simulink model "Quadcopter_State_model_Arduino"  (R2023b)
settings: Solver=VariableStepAuto  StartTime=0.0  StopTime=inf  FixedStep=0.00001  MinStep=0.001  RelTol=1e-3
model workspace (MAT data in the model file):
  DesiredPitchRoll : sugfis (value not decoded)
  DesiredThrust : sugfis (value not decoded)
  DesiredYaw : sugfis (value not decoded)
  Desired_Pitch = 0
  Desired_Roll = 0
  Desired_Yaw = 0
  Desired_Z_Velocity = -3
  FuzzyMotorspeed : sugfis (value not decoded)
values from neighbouring files (symbols this model uses):
  g = 9.81    [Quadcopter_Constants.m]
  Ixx = 0.0294838    [Quadcopter_Constants.m]
  Iyy = 0.0294838    [Quadcopter_Constants.m]
  Izz = 0.058967624    [Quadcopter_Constants.m]
  Jr = (6e-5)*1.358    (= 8.148e-05)    [Quadcopter_Constants.m]
  kd = 1    [Quadcopter_Constants.m]
  kd_phi = 1    [Quadcopter_Constants.m]
  kd_theta = 1    [Quadcopter_Constants.m]
  kf = 1    [Quadcopter_Constants.m]
  ki = 1    [Quadcopter_Constants.m]
  ki_phi = 1    [Quadcopter_Constants.m]
  ki_theta = 1    [Quadcopter_Constants.m]
  km = 4.74157e-9    (= 4.74157e-09)    [Quadcopter_Constants.m]
  kp = 1    [Quadcopter_Constants.m]
  kp_phi = 1    [Quadcopter_Constants.m]
  kp_theta = 1    [Quadcopter_Constants.m]
  kr = (0.1)*1.358    (= 0.1358)    [Quadcopter_Constants.m]
  kt = (0.1)*1.358    (= 0.1358)    [Quadcopter_Constants.m]
  l = 0.254    [Quadcopter_Constants.m]
  m = 0.914    [Quadcopter_Constants.m]
  sample_freq = 1000    [Quadcopter_Constants.m]
undefined symbols (not defined in the file or in its folder): LF
libraries: fuzblock x18, instrumentseriallib x12, simulink_extras x6, vrlib x4, instrumentlib x3, etargetslib x1, slpidlib x1, simulink x1
(part 3 of 5)

== system Quadcopter_State_model_Arduino/Arduino Sim/Control Vector ==
  Omega_1 : Inport
  Omega_2 : Inport  Port=2
  Omega_3 : Inport  Port=3
  Omega_4 : Inport  Port=4
  Constant : Constant  Value=kf
  Constant1 : Constant  Value=km
  Product{,1..3} (4 alike) : Product
  Square{,1..3} (4 alike) : Math  Operator=square
  Sum : Sum  Inputs=++++
  Sum1 : Sum  Inputs=-+
  Sum2 : Sum  Inputs=+-
  Sum3 : Sum  Inputs=+-+-
  U1 : Outport
  U2 : Outport  Port=2
  U3 : Outport  Port=3
  U4 : Outport  Port=4
  wires:
  Omega_1/1 -> Square/1
  Omega_2/1 -> Square1/1
  Omega_3/1 -> Square2/1
  Omega_4/1 -> Square3/1
  Constant/1 -> Product2/2, Product1/2, Product/2
  Sum/1 -> Product/1
  Product/1 -> U1/1
  Square/1 -> Sum3/1, Sum2/1, Sum/1
  Square1/1 -> Sum3/2, Sum1/1, Sum/2
  Square2/1 -> Sum3/3, Sum2/2, Sum/3
  Square3/1 -> Sum1/2, Sum/4, Sum3/4
  Sum1/1 -> Product1/1
  Product1/1 -> U2/1
  Sum2/1 -> Product2/1
  Product2/1 -> U3/1
  Constant1/1 -> Product3/2
  Sum3/1 -> Product3/1
  Product3/1 -> U4/1

== system Quadcopter_State_model_Arduino/Arduino Sim/Quadcopter Dynamics1 ==
  U1 : Inport
  U2 : Inport  Port=2
  U3 : Inport  Port=3
  U4 : Inport  Port=4
  Omega_R : Inport  Port=5
  Bus Creator : BusCreator  Inputs=12
  Rotational Subsystem : Subsystem
  Translational Subsystem 2.0 : Subsystem
  Translational Wind Engine : Subsystem
  X_State : Outport
  wires:
  Rotational Subsystem/5(psi) -> Translational Subsystem 2.0/4(psi), Translational Wind Engine/3(psi), Bus Creator/5  "psi"
  Rotational Subsystem/2(phi_dot) -> Bus Creator/2  "phi_dot"
  Rotational Subsystem/3(theta) -> Translational Subsystem 2.0/3(theta), Translational Wind Engine/2(theta), Bus Creator/3  "theta"
  Rotational Subsystem/1(phi) -> Translational Subsystem 2.0/2(phi), Translational Wind Engine/1(phi), Bus Creator/1  "phi"
  Rotational Subsystem/4(theta_dot) -> Bus Creator/4  "theta_dot"
  Bus Creator/1 -> X_State/1  "X_State"
  Rotational Subsystem/6(psi_dot) -> Bus Creator/6  "psi_dot"
  U4/1 -> Rotational Subsystem/3(U4)
  U3/1 -> Rotational Subsystem/2(U3)
  U2/1 -> Rotational Subsystem/1(U2)
  Omega_R/1 -> Rotational Subsystem/4(Omega_R)
  Translational Wind Engine/1(FWx) -> Translational Subsystem 2.0/5(FWx)
  Translational Wind Engine/2(FWy) -> Translational Subsystem 2.0/6(FWy)
  Translational Wind Engine/3(FWz) -> Translational Subsystem 2.0/7(FWz)
  U1/1 -> Translational Subsystem 2.0/1(U1)
  Translational Subsystem 2.0/1(x) -> Bus Creator/7  "x"
  Translational Subsystem 2.0/2(x_dot) -> Bus Creator/8  "x_dot"
  Translational Subsystem 2.0/3(y) -> Bus Creator/9  "y"
  Translational Subsystem 2.0/4(y_dot) -> Bus Creator/10  "y_dot"
  Translational Subsystem 2.0/5(z) -> Bus Creator/11  "z"
  Translational Subsystem 2.0/6(z_dot) -> Bus Creator/12  "z_dot"

== system Quadcopter_State_model_Arduino/Arduino Sim/Relative Speed ==
  Omega_1 : Inport
  Omega_2 : Inport  Port=2
  Omega_3 : Inport  Port=3
  Omega_4 : Inport  Port=4
  Add4 : Sum  Inputs=-+-+
  Omega_R : Outport
  wires:
  Omega_1/1 -> Add4/1
  Add4/1 -> Omega_R/1  "Omega_R"
  Omega_2/1 -> Add4/2
  Omega_3/1 -> Add4/3
  Omega_4/1 -> Add4/4

== system Quadcopter_State_model_Arduino/Arduino Sim/Visualization ==
  X_State : Inport
  Bus Creator1 : BusCreator  Inputs=3
  Bus Selector1 : BusSelector  OutputSignals=phi,phi_dot,theta,theta_dot,psi,psi_dot,x,x_dot,y,y_dot,z,z_dot
  Gain : Gain
  Gain1 : Gain  Gain=-1
  Gain2 : Gain
  Gain3 : Gain  Gain=-1
  Gain4 : Gain  Gain=-1
  Inertal to body frame : MATLAB Function  TreatAsAtomicUnit=on
  Rotation Matrix to VRML Rotation1 : vrlib/Utilities/Rotation Matrix to VR Rotation  maxzero=1e-12
  VR Sink : vrlib/VR Sink  InstantiateOnLoad=on  SampleTime=0.1  ViewEnable=on  RemoteChange=off  RemoteView=off  FieldsWritten=Wall_Mat.diffuseColor.3.1.1.double#Window_Mat.transparency.1.1.1.double#Landing_Mat.diffuseColor.3.1.1.double#Pole_1.Color.3.1.1.double#UAV.rotation.4.1.1.double#UAV.translation.3.1.1.double#HUDText1.string.1.-1.1.char  WorldFileName=uav_scene_drone_example.wrl  WorldDescription=UAV Competition Scene  AutoView=off  VideoDimensions=[]  AllowVariableSize=off  FigureProperties=[]
  wires:
  Bus Selector1/4 -> ?  "<theta_dot>"
  Bus Selector1/10 -> ?  "<y_dot>"
  X_State/1 -> Bus Selector1/1
  Bus Creator1/1 -> VR Sink/6  "X_State"
  Bus Selector1/2 -> ?  "<phi_dot>"
  Inertal to body frame/1(R) -> Rotation Matrix to VRML Rotation1/1
  ? -> VR Sink/7
  Rotation Matrix to VRML Rotation1/1 -> VR Sink/5
  ? -> VR Sink/4
  Bus Selector1/6 -> ?  "<psi_dot>"
  Bus Selector1/8 -> ?  "<x_dot>"
  Bus Selector1/12 -> ?  "<z_dot>"
  ? -> VR Sink/1
  ? -> VR Sink/2
  ? -> VR Sink/3
  Bus Selector1/11 -> Gain1/1  "<z>"
  Bus Selector1/9 -> Gain/1  "<y>"
  Bus Selector1/3 -> Gain3/1  "<theta>"
  Bus Selector1/5 -> Gain4/1  "<psi>"
  Bus Selector1/1 -> Inertal to body frame/3(psi)  "<phi>"
  Gain/1 -> Bus Creator1/1
  Gain1/1 -> Bus Creator1/2
  Bus Selector1/7 -> Gain2/1  "<x>"
  Gain2/1 -> Bus Creator1/3
  Gain3/1 -> Inertal to body frame/1(phi)
  Gain4/1 -> Inertal to body frame/2(theta)

== system Quadcopter_State_model_Arduino/Board Fuzzy Only/Control Vector ==
  Omega_1 : Inport
  Omega_2 : Inport  Port=2
  Omega_3 : Inport  Port=3
  Omega_4 : Inport  Port=4
  Constant : Constant  Value=kf
  Constant1 : Constant  Value=km
  Product{,1..3} (4 alike) : Product
  Square{,1..3} (4 alike) : Math  Operator=square
  Sum : Sum  Inputs=++++
  Sum1 : Sum  Inputs=-+
  Sum2 : Sum  Inputs=+-
  Sum3 : Sum  Inputs=+-+-
  U1 : Outport
  U2 : Outport  Port=2
  U3 : Outport  Port=3
  U4 : Outport  Port=4
  wires:
  Omega_1/1 -> Square/1
  Omega_2/1 -> Square1/1
  Omega_3/1 -> Square2/1
  Omega_4/1 -> Square3/1
  Constant/1 -> Product2/2, Product1/2, Product/2
  Sum/1 -> Product/1
  Product/1 -> U1/1
  Square/1 -> Sum3/1, Sum2/1, Sum/1
  Square1/1 -> Sum3/2, Sum1/1, Sum/2
  Square2/1 -> Sum3/3, Sum2/2, Sum/3
  Square3/1 -> Sum1/2, Sum/4, Sum3/4
  Sum1/1 -> Product1/1
  Product1/1 -> U2/1
  Sum2/1 -> Product2/1
  Product2/1 -> U3/1
  Constant1/1 -> Product3/2
  Sum3/1 -> Product3/1
  Product3/1 -> U4/1

== system Quadcopter_State_model_Arduino/Board Fuzzy Only/Fuzzy Control System ==
  note: Outputs are also mapped to a unsigned
      | 8-bit integer range. [0,255] This can be
      | scaled with a gain block or my changing
      | the FIS parameters.
  note: Here the inputs are mapped to an 8-bit integer currently.
      | Thrust: [0,255]
      | Roll: [-128,127]
      | Pitch: [-128,127]
      | Yaw: [-128,127]
      | While these are controlled by sliders currently they
      | could be controlled by a user using twin analog joysticks
      | or by another intelligent system directing flight.
      | To make a system that balances itself we could use
      | readings off the 9-axis gyro to inform the system to
      | lean in the opposite direction.
  x_state : Inport
  Attitude Controller : Subsystem
  Bus Creator : BusCreator  Inputs=4
  Bus Selector1 : BusSelector  OutputSignals=phi,phi_dot,theta,theta_dot,psi,psi_dot,x,x_dot,y,y_dot,z,z_dot
  Heading Controller : Subsystem
  Motorspeeds : fuzblock/Fuzzy Logic  Controller  FIS=FuzzyMotorspeed  OutputSampleNumber=101  DataType=double  FuzzifiedInputs=off  RuleFiringStrengths=off  RuleOutputs=off  AggregatedOutputs=off  SimulateUsing=Interpreted execution  OutOfRangeInputValueMessage=warning  NoRuleFiredMessage=warning  EmptyOutputFuzzySetMessage=warning
  Saturation1 : Saturate  UpperLimit=255  LowerLimit=0  OutMin=[0]  OutMax=[255]
  Scope4 : Scope  NumInputPorts=4
  Thrust Controller : Subsystem
  motorspeeds : Outport
  wires:
  Motorspeeds/1 -> motorspeeds/1
  Bus Selector1/9 -> ?  "<y>"
  Bus Creator/1 -> Motorspeeds/1
  Bus Selector1/8 -> ?  "<x_dot>"
  x_state/1 -> Bus Selector1/1
  Bus Selector1/7 -> ?  "<x>"
  Bus Selector1/10 -> ?  "<y_dot>"
  Bus Selector1/11 -> ?  "<z>"
  Attitude Controller/1(Desired Roll1) -> Bus Creator/2, Scope4/2  "Desired Roll"
  Attitude Controller/2(Desired Pitch1) -> Scope4/3, Bus Creator/3  "Desired Pitch"
  Bus Selector1/1 -> Attitude Controller/1(<phi>)  "<phi>"
  Bus Selector1/2 -> Attitude Controller/2(<phi_dot>)  "<phi_dot>"
  Bus Selector1/3 -> Attitude Controller/3(<theta>)  "<theta>"
  Bus Selector1/4 -> Attitude Controller/4(<theta_dot>)  "<theta_dot>"
  Heading Controller/1(Desired Yaw1) -> Bus Creator/4, Scope4/4
  Bus Selector1/5 -> Heading Controller/1(<psi>)  "<psi>"
  Bus Selector1/6 -> Heading Controller/2(<psi_dot>)  "<psi_dot>"
  Bus Selector1/12 -> Thrust Controller/1(<z_dot>)  "<z_dot>"
  Thrust Controller/1(Desired Thrust1) -> Scope4/1, Bus Creator/1

== system Quadcopter_State_model_Arduino/Board Fuzzy Only/Fuzzy Control System1 ==
  note: Outputs are also mapped to a unsigned
      | 8-bit integer range. [0,255] This can be
      | scaled with a gain block or my changing
      | the FIS parameters.
  note: Here the inputs are mapped to an 8-bit integer currently.
      | Thrust: [0,255]
      | Roll: [-128,127]
      | Pitch: [-128,127]
      | Yaw: [-128,127]
      | While these are controlled by sliders currently they
      | could be controlled by a user using twin analog joysticks
      | or by another intelligent system directing flight.
      | To make a system that balances itself we could use
      | readings off the 9-axis gyro to inform the system to
      | lean in the opposite direction.
  x_state : Inport
  Attitude Controller : Subsystem
  Bus Selector1 : BusSelector  OutputSignals=phi,phi_dot,theta,theta_dot,psi,psi_dot,x,x_dot,y,y_dot,z,z_dot
  Heading Controller : Subsystem
  MMA : Subsystem
  Saturation1 : Saturate  UpperLimit=255  LowerLimit=0  OutMin=[0]  OutMax=[255]
  Scope4 : Scope  NumInputPorts=4
  Thrust Controller : Subsystem
  motorspeeds : Outport
  wires:
  MMA/1(motorspeeds) -> motorspeeds/1
  Bus Selector1/9 -> ?  "<y>"
  Bus Selector1/8 -> ?  "<x_dot>"
  x_state/1 -> Bus Selector1/1
  Bus Selector1/7 -> ?  "<x>"
  Bus Selector1/10 -> ?  "<y_dot>"
  Bus Selector1/11 -> ?  "<z>"
  Attitude Controller/1(Desired Roll1) -> MMA/4(Desired Roll1), Scope4/2  "Desired Roll"
  Attitude Controller/2(Desired Pitch1) -> MMA/3(Desired Pitch1), Scope4/3  "Desired Pitch"
  Bus Selector1/1 -> Attitude Controller/1(<phi>)  "<phi>"
  Bus Selector1/2 -> Attitude Controller/2(<phi_dot>)  "<phi_dot>"
  Bus Selector1/3 -> Attitude Controller/3(<theta>)  "<theta>"
  Bus Selector1/4 -> Attitude Controller/4(<theta_dot>)  "<theta_dot>"
  Heading Controller/1(Desired Yaw1) -> MMA/2(Desired Yaw1), Scope4/4
  Bus Selector1/5 -> Heading Controller/1(<psi>)  "<psi>"
  Bus Selector1/6 -> Heading Controller/2(<psi_dot>)  "<psi_dot>"
  Bus Selector1/12 -> Thrust Controller/1(<z_dot>)  "<z_dot>"
  Thrust Controller/1(Desired Thrust1) -> MMA/1(Desired Thrust1), Scope4/1

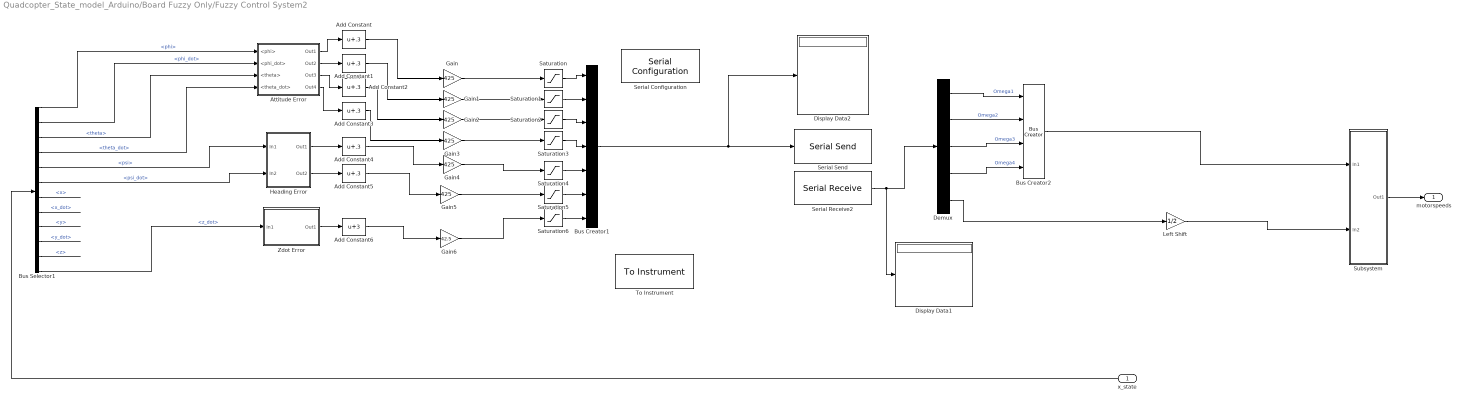
== system Quadcopter_State_model_Arduino/Board Fuzzy Only/Fuzzy Control System2 ==
  x_state : Inport
  Add Constant{,1..5} (6 alike) : Bias  Bias=.3  SaturateOnIntegerOverflow=off
  Add Constant6 : Bias  Bias=3  SaturateOnIntegerOverflow=off
  Attitude Error : Subsystem
  Bus Creator1 : BusCreator  Inputs=7
  Bus Creator2 : BusCreator  Inputs=4
  Bus Selector1 : BusSelector  OutputSignals=phi,phi_dot,theta,theta_dot,psi,psi_dot,x,x_dot,y,y_dot,z,z_dot
  Demux : Demux  Outputs=5
  Display Data1 : Display
  Display Data2 : Display
  Gain{,1..5} (6 alike) : Gain  Gain=425
  Gain6 : Gain  Gain=42.5
  Heading Error : Subsystem
  Left Shift : Gain  Gain=1/2
  Saturation{,1..6} (7 alike) : Saturate  UpperLimit=255  LowerLimit=0
  Serial Configuration : instrumentseriallib/Serial Configuration  Priority=-200000  PortSel=COM8  Port=COM8  ComPort=COM8  BaudRate=9600  DataBits=8  Parity=none  StopBits=1  ByteOrder=little-endian  FlowControl=none  Timeout=10  SimulateUsing=Interpreted execution  BlockInModel=on  aMode=1
  Serial Receive2 : instrumentseriallib/Serial Receive  Priority=1  PortSel=COM8  Port=COM8  ComPort=COM8  DataType=uint8  SaveDataType=uint8  ToggleHeader=off  Header=[]  ToggleTerminator=off  Terminator=LF ('\n')  CustomTerminator=[]  InputFormat=Column major  ToggleDataSize=on  DataSize=[1 5]  EnableBlockingMode=on  ActionDataUnavailable=Output custom value  ActionWhenDataUnavailable=Output custom value  CustomValue=[127 127 127 127 127]  SampleTime=0.01  SimulateUsing=Interpreted execution  BlockInModel=on  aMode=1
  Serial Send : instrumentseriallib/Serial Send  Priority=1  PortSel=COM8  Port=COM8  ComPort=COM8  Header=[]  Terminator=<none>  CustomTerminator=[]  EnableBlockingMode=on  SimulateUsing=Interpreted execution  BlockInModel=on  aMode=1
  Subsystem : Subsystem
  To Instrument : instrumentlib/To Instrument  sampleTime=-1  isWorkspaceObject=off  timeout=10  inputBufferSize=8192  protocol=Serial  serialPort=COM1  baudRate=9600  gpibVendor=ICS Electronics  boardIndex=0  primaryAddress=1  secondaryAddress=0  visaVendor=Keysight  visaSerialPort=0  chassisIndex=0  logicalAddress=0  tcpRemoteHost='127.0.0.1'  tcpRemotePort=4500  udpRemoteHost='127.0.0.1'  udpRemotePort=9090  visaTCPBoardIndex=0  visaTCPRemoteHost='127.0.0.1'  usbBoardIndex=0  usbManufID=0  usbModelCode=0  usbSerialNumber=0  initAction=None  initCommand='DATA:SOURCE CH1'  initFunction=get  command=''  sendFormat=ASCII  asciiFormatting='%d'  precision=8-bit integer  byteOrder=Little endian
  Zdot Error : Subsystem
  motorspeeds : Outport
  wires:
  Bus Selector1/9 -> ?  "<y>"
  Bus Selector1/8 -> ?  "<x_dot>"
  x_state/1 -> Bus Selector1/1
  Bus Selector1/7 -> ?  "<x>"
  Bus Selector1/10 -> ?  "<y_dot>"
  Bus Selector1/11 -> ?  "<z>"
  Bus Selector1/5 -> Heading Error/1(In1)  "<psi>"
  Bus Selector1/6 -> Heading Error/2(In2)  "<psi_dot>"
  Bus Selector1/12 -> Zdot Error/1(In1)  "<z_dot>"
  Demux/5 -> Left Shift/1
  Bus Creator2/1 -> Subsystem/1(In1)
  Subsystem/1(Out1) -> motorspeeds/1
  Bus Selector1/1 -> Attitude Error/1(<phi>)  "<phi>"
  Bus Selector1/2 -> Attitude Error/2(<phi_dot>)  "<phi_dot>"
  Bus Selector1/3 -> Attitude Error/3(<theta>)  "<theta>"
  Bus Selector1/4 -> Attitude Error/4(<theta_dot>)  "<theta_dot>"
  Attitude Error/1(Out1) -> Add Constant/1
  Attitude Error/2(Out2) -> Add Constant1/1
  Attitude Error/3(Out3) -> Add Constant2/1
  Attitude Error/4(Out4) -> Add Constant3/1
  Saturation/1 -> Bus Creator1/1
  Saturation1/1 -> Bus Creator1/2
  Saturation2/1 -> Bus Creator1/3
  Saturation3/1 -> Bus Creator1/4
  Add Constant/1 -> Gain/1
  Add Constant1/1 -> Gain1/1
  Add Constant2/1 -> Gain2/1
  Add Constant3/1 -> Gain3/1
  Saturation4/1 -> Bus Creator1/5
  Saturation5/1 -> Bus Creator1/6
  Saturation6/1 -> Bus Creator1/7
  Gain/1 -> Saturation/1
  Gain1/1 -> Saturation1/1
  Gain2/1 -> Saturation2/1
  Gain3/1 -> Saturation3/1
  Heading Error/1(Out1) -> Add Constant4/1
  Heading Error/2(Out2) -> Add Constant5/1
  Add Constant5/1 -> Gain5/1
  Add Constant4/1 -> Gain4/1
  Gain5/1 -> Saturation5/1
  Gain4/1 -> Saturation4/1
  Zdot Error/1(Out1) -> Add Constant6/1
  Add Constant6/1 -> Gain6/1
  Gain6/1 -> Saturation6/1
  Demux/1 -> Bus Creator2/1  "Omega1"
  Demux/2 -> Bus Creator2/2  "Omega2"
  Demux/3 -> Bus Creator2/3  "Omega3"
  Demux/4 -> Bus Creator2/4  "Omega4"
  Left Shift/1 -> Subsystem/2(In2)
  Serial Receive2/1 -> Display Data1/1, Demux/1
  Bus Creator1/1 -> Display Data2/1, Serial Send/1

== system Quadcopter_State_model_Arduino/Board Fuzzy Only/Quadcopter Dynamics1 ==
  U1 : Inport
  U2 : Inport  Port=2
  U3 : Inport  Port=3
  U4 : Inport  Port=4
  Omega_R : Inport  Port=5
  Bus Creator : BusCreator  Inputs=12
  Rotational Subsystem : Subsystem
  Translational Subsystem 2.0 : Subsystem
  Translational Wind Engine : Subsystem
  X_State : Outport
  wires:
  Rotational Subsystem/5(psi) -> Translational Subsystem 2.0/4(psi), Translational Wind Engine/3(psi), Bus Creator/5  "psi"
  Rotational Subsystem/2(phi_dot) -> Bus Creator/2  "phi_dot"
  Rotational Subsystem/3(theta) -> Translational Subsystem 2.0/3(theta), Translational Wind Engine/2(theta), Bus Creator/3  "theta"
  Rotational Subsystem/1(phi) -> Translational Subsystem 2.0/2(phi), Translational Wind Engine/1(phi), Bus Creator/1  "phi"
  Rotational Subsystem/4(theta_dot) -> Bus Creator/4  "theta_dot"
  Bus Creator/1 -> X_State/1  "X_State"
  Rotational Subsystem/6(psi_dot) -> Bus Creator/6  "psi_dot"
  U4/1 -> Rotational Subsystem/3(U4)
  U3/1 -> Rotational Subsystem/2(U3)
  U2/1 -> Rotational Subsystem/1(U2)
  Omega_R/1 -> Rotational Subsystem/4(Omega_R)
  Translational Wind Engine/1(FWx) -> Translational Subsystem 2.0/5(FWx)
  Translational Wind Engine/2(FWy) -> Translational Subsystem 2.0/6(FWy)
  Translational Wind Engine/3(FWz) -> Translational Subsystem 2.0/7(FWz)
  U1/1 -> Translational Subsystem 2.0/1(U1)
  Translational Subsystem 2.0/1(x) -> Bus Creator/7  "x"
  Translational Subsystem 2.0/2(x_dot) -> Bus Creator/8  "x_dot"
  Translational Subsystem 2.0/3(y) -> Bus Creator/9  "y"
  Translational Subsystem 2.0/4(y_dot) -> Bus Creator/10  "y_dot"
  Translational Subsystem 2.0/5(z) -> Bus Creator/11  "z"
  Translational Subsystem 2.0/6(z_dot) -> Bus Creator/12  "z_dot"

== system Quadcopter_State_model_Arduino/Board Fuzzy Only/Relative Speed ==
  Omega_1 : Inport
  Omega_2 : Inport  Port=2
  Omega_3 : Inport  Port=3
  Omega_4 : Inport  Port=4
  Add4 : Sum  Inputs=-+-+
  Omega_R : Outport
  wires:
  Omega_1/1 -> Add4/1
  Add4/1 -> Omega_R/1  "Omega_R"
  Omega_2/1 -> Add4/2
  Omega_3/1 -> Add4/3
  Omega_4/1 -> Add4/4

== system Quadcopter_State_model_Arduino/Fuzzy Simulation/Arduino Communication ==
  X_State : Inport
  Bus Selector : BusSelector  OutputSignals=theta,phi,psi,z_dot,theta_dot,phi_dot,psi_dot
  Cast To Single{,1..6} (7 alike) : DataTypeConversion  OutDataTypeStr=single  SaturateOnIntegerOverflow=off  RndMeth=Floor
  Desired Pitch : Constant  Value=-1  OutDataTypeStr=single
  Desired Roll : Constant  Value=-1  OutDataTypeStr=single
  Desired Yaw : Constant  Value=-1  OutDataTypeStr=single
  Desired Z Velocity : Constant  Value=-1  OutDataTypeStr=single
  Display : Display
  Display1 : Display
  Gain : Gain  Gain=pi  OutDataTypeStr=single
  Gain1 : Gain  Gain=pi  OutDataTypeStr=single
  Gain2 : Gain  Gain=pi  OutDataTypeStr=single
  MATLAB Function : MATLAB Function  TreatAsAtomicUnit=on
  Matrix Concatenate : Concatenate  NumInputs=11  ConcatenateDimension=2
  Radians to Degrees : simulink_extras/Transformations/Radians to Degrees
  Radians to Degrees1 : simulink_extras/Transformations/Radians to Degrees
  Radians to Degrees2 : simulink_extras/Transformations/Radians to Degrees
  Serial Configuration : instrumentseriallib/Serial Configuration  Priority=-200000  PortSel=COM15  Port=COM15  ComPort=COM15  BaudRate=9600  DataBits=8  Parity=none  StopBits=1  ByteOrder=little-endian  FlowControl=none  Timeout=10  SimulateUsing=Interpreted execution  BlockInModel=on  aMode=1
  Serial Receive : instrumentseriallib/Serial Receive  Priority=1  PortSel=COM15  Port=COM15  ComPort=COM15  DataType=uint8  SaveDataType=uint8  ToggleHeader=off  Header=[]  ToggleTerminator=off  Terminator=<none>  CustomTerminator=[]  InputFormat=Column major  ToggleDataSize=on  DataSize=[1 4]  EnableBlockingMode=on  ActionDataUnavailable=Output last received value  ActionWhenDataUnavailable=Output last received value  CustomValue=0  SampleTime=0.01  SimulateUsing=Interpreted execution  BlockInModel=on  aMode=1
  Serial Send : instrumentseriallib/Serial Send  Priority=1  PortSel=COM15  Port=COM15  ComPort=COM15  Header=[]  Terminator=<none>  CustomTerminator=[]  EnableBlockingMode=on  SimulateUsing=Interpreted execution  BlockInModel=on  aMode=1
  Sin : Trigonometry
  Sin1 : Trigonometry
  Sin2 : Trigonometry
  Omega_1 : Outport
  Omega_2 : Outport  Port=2
  Omega_3 : Outport  Port=3
  Omega_4 : Outport  Port=4
  wires:
  X_State/1 -> Bus Selector/1
  Bus Selector/2 -> Cast To Single5/1  "<phi>"
  Bus Selector/4 -> Cast To Single/1  "<z_dot>"
  Bus Selector/3 -> Cast To Single6/1  "<psi>"
  Radians to Degrees/1 -> Matrix Concatenate/1  "roll_meas"
  Radians to Degrees1/1 -> Matrix Concatenate/2  "pitch_meas"
  Radians to Degrees2/1 -> Matrix Concatenate/3  "yaw_meas"
  Bus Selector/5 -> Cast To Single1/1  "<theta_dot>"
  Bus Selector/6 -> Cast To Single2/1  "<phi_dot>"
  Bus Selector/7 -> Cast To Single3/1  "<psi_dot>"
  Bus Selector/1 -> Cast To Single4/1  "<theta>"
  Sin/1 -> Gain/1
  Gain/1 -> Radians to Degrees/1
  Gain1/1 -> Radians to Degrees1/1
  Sin1/1 -> Gain1/1
  Gain2/1 -> Radians to Degrees2/1
  Sin2/1 -> Gain2/1
  MATLAB Function/1(m1o) -> Omega_1/1
  MATLAB Function/2(m2o) -> Omega_2/1
  MATLAB Function/3(m3o) -> Omega_3/1
  MATLAB Function/4(m4o) -> Omega_4/1
  Desired Yaw/1 -> Matrix Concatenate/10  "inputYaw"
  Desired Z Velocity/1 -> Matrix Concatenate/11  "inputZdot"
  Desired Pitch/1 -> Matrix Concatenate/9  "inputPitch"
  Desired Roll/1 -> Matrix Concatenate/8  "inputRoll"
  Matrix Concatenate/1 -> Display1/1, Serial Send/1
  Serial Receive/1 -> Display/1, MATLAB Function/1(m)
  Cast To Single/1 -> Matrix Concatenate/4
  Cast To Single1/1 -> Matrix Concatenate/5
  Cast To Single2/1 -> Matrix Concatenate/6
  Cast To Single3/1 -> Matrix Concatenate/7
  Cast To Single4/1 -> Sin/1
  Cast To Single5/1 -> Sin1/1
  Cast To Single6/1 -> Sin2/1

== system Quadcopter_State_model_Arduino/Fuzzy Simulation/Control Vector ==
  Omega_1 : Inport
  Omega_2 : Inport  Port=2
  Omega_3 : Inport  Port=3
  Omega_4 : Inport  Port=4
  Constant : Constant  Value=kf
  Constant1 : Constant  Value=km
  Product{,1..3} (4 alike) : Product
  Square{,1..3} (4 alike) : Math  Operator=square
  Sum : Sum  Inputs=++++
  Sum1 : Sum  Inputs=-+
  Sum2 : Sum  Inputs=+-
  Sum3 : Sum  Inputs=+-+-
  U1 : Outport
  U2 : Outport  Port=2
  U3 : Outport  Port=3
  U4 : Outport  Port=4
  wires:
  Omega_1/1 -> Square/1
  Omega_2/1 -> Square1/1
  Omega_3/1 -> Square2/1
  Omega_4/1 -> Square3/1
  Constant/1 -> Product2/2, Product1/2, Product/2
  Sum/1 -> Product/1
  Product/1 -> U1/1
  Square/1 -> Sum3/1, Sum2/1, Sum/1
  Square1/1 -> Sum3/2, Sum1/1, Sum/2
  Square2/1 -> Sum3/3, Sum2/2, Sum/3
  Square3/1 -> Sum1/2, Sum/4, Sum3/4
  Sum1/1 -> Product1/1
  Product1/1 -> U2/1
  Sum2/1 -> Product2/1
  Product2/1 -> U3/1
  Constant1/1 -> Product3/2
  Sum3/1 -> Product3/1
  Product3/1 -> U4/1

== system Quadcopter_State_model_Arduino/Fuzzy Simulation/Fuzzy Control System ==
  note: Outputs are also mapped to a unsigned
      | 8-bit integer range. [0,255] This can be
      | scaled with a gain block or my changing
      | the FIS parameters.
  note: Here the inputs are mapped to an 8-bit integer currently.
      | Thrust: [0,255]
      | Roll: [-128,127]
      | Pitch: [-128,127]
      | Yaw: [-128,127]
      | While these are controlled by sliders currently they
      | could be controlled by a user using twin analog joysticks
      | or by another intelligent system directing flight.
      | To make a system that balances itself we could use
      | readings off the 9-axis gyro to inform the system to
      | lean in the opposite direction.
  x_state : Inport
  Attitude Controller : Subsystem
  Bus Creator : BusCreator  Inputs=4
  Bus Selector1 : BusSelector  OutputSignals=phi,phi_dot,theta,theta_dot,psi,psi_dot,x,x_dot,y,y_dot,z,z_dot
  Heading Controller : Subsystem
  Motorspeeds : fuzblock/Fuzzy Logic  Controller  FIS=FuzzyMotorspeed  OutputSampleNumber=101  DataType=double  FuzzifiedInputs=off  RuleFiringStrengths=off  RuleOutputs=off  AggregatedOutputs=off  SimulateUsing=Interpreted execution  OutOfRangeInputValueMessage=warning  NoRuleFiredMessage=warning  EmptyOutputFuzzySetMessage=warning
  Saturation1 : Saturate  UpperLimit=255  LowerLimit=0  OutMin=[0]  OutMax=[255]
  Scope4 : Scope  NumInputPorts=4
  Thrust Controller : Subsystem
  motorspeeds : Outport
  wires:
  Motorspeeds/1 -> motorspeeds/1
  Bus Selector1/9 -> ?  "<y>"
  Bus Creator/1 -> Motorspeeds/1
  Bus Selector1/8 -> ?  "<x_dot>"
  x_state/1 -> Bus Selector1/1
  Bus Selector1/7 -> ?  "<x>"
  Bus Selector1/10 -> ?  "<y_dot>"
  Bus Selector1/11 -> ?  "<z>"
  Attitude Controller/1(Desired Roll1) -> Bus Creator/2, Scope4/2  "Desired Roll"
  Attitude Controller/2(Desired Pitch1) -> Scope4/3, Bus Creator/3  "Desired Pitch"
  Bus Selector1/1 -> Attitude Controller/1(<phi>)  "<phi>"
  Bus Selector1/2 -> Attitude Controller/2(<phi_dot>)  "<phi_dot>"
  Bus Selector1/3 -> Attitude Controller/3(<theta>)  "<theta>"
  Bus Selector1/4 -> Attitude Controller/4(<theta_dot>)  "<theta_dot>"
  Heading Controller/1(Desired Yaw1) -> Bus Creator/4, Scope4/4
  Bus Selector1/5 -> Heading Controller/1(<psi>)  "<psi>"
  Bus Selector1/6 -> Heading Controller/2(<psi_dot>)  "<psi_dot>"
  Bus Selector1/12 -> Thrust Controller/1(<z_dot>)  "<z_dot>"
  Thrust Controller/1(Desired Thrust1) -> Scope4/1, Bus Creator/1

== system Quadcopter_State_model_Arduino/Fuzzy Simulation/Fuzzy Control System1 ==
  note: Outputs are also mapped to a unsigned
      | 8-bit integer range. [0,255] This can be
      | scaled with a gain block or my changing
      | the FIS parameters.
  note: Here the inputs are mapped to an 8-bit integer currently.
      | Thrust: [0,255]
      | Roll: [-128,127]
      | Pitch: [-128,127]
      | Yaw: [-128,127]
      | While these are controlled by sliders currently they
      | could be controlled by a user using twin analog joysticks
      | or by another intelligent system directing flight.
      | To make a system that balances itself we could use
      | readings off the 9-axis gyro to inform the system to
      | lean in the opposite direction.
  x_state : Inport
  Attitude Controller : Subsystem
  Bus Selector1 : BusSelector  OutputSignals=phi,phi_dot,theta,theta_dot,psi,psi_dot,x,x_dot,y,y_dot,z,z_dot
  Heading Controller : Subsystem
  MMA : Subsystem
  Saturation1 : Saturate  UpperLimit=255  LowerLimit=0  OutMin=[0]  OutMax=[255]
  Scope4 : Scope  NumInputPorts=4
  Thrust Controller : Subsystem
  motorspeeds : Outport
  wires:
  MMA/1(motorspeeds) -> motorspeeds/1
  Bus Selector1/9 -> ?  "<y>"
  Bus Selector1/8 -> ?  "<x_dot>"
  x_state/1 -> Bus Selector1/1
  Bus Selector1/7 -> ?  "<x>"
  Bus Selector1/10 -> ?  "<y_dot>"
  Bus Selector1/11 -> ?  "<z>"
  Attitude Controller/1(Desired Roll1) -> MMA/4(Desired Roll1), Scope4/2  "Desired Roll"
  Attitude Controller/2(Desired Pitch1) -> MMA/3(Desired Pitch1), Scope4/3  "Desired Pitch"
  Bus Selector1/1 -> Attitude Controller/1(<phi>)  "<phi>"
  Bus Selector1/2 -> Attitude Controller/2(<phi_dot>)  "<phi_dot>"
  Bus Selector1/3 -> Attitude Controller/3(<theta>)  "<theta>"
  Bus Selector1/4 -> Attitude Controller/4(<theta_dot>)  "<theta_dot>"
  Heading Controller/1(Desired Yaw1) -> MMA/2(Desired Yaw1), Scope4/4
  Bus Selector1/5 -> Heading Controller/1(<psi>)  "<psi>"
  Bus Selector1/6 -> Heading Controller/2(<psi_dot>)  "<psi_dot>"
  Bus Selector1/12 -> Thrust Controller/1(<z_dot>)  "<z_dot>"
  Thrust Controller/1(Desired Thrust1) -> MMA/1(Desired Thrust1), Scope4/1

== system Quadcopter_State_model_Arduino/Fuzzy Simulation/Fuzzy Control System2 ==
  note: Outputs are also mapped to a unsigned
      | 8-bit integer range. [0,255] This can be
      | scaled with a gain block or my changing
      | the FIS parameters.
  note: Here the inputs are mapped to an 8-bit integer currently.
      | Thrust: [0,255]
      | Roll: [-128,127]
      | Pitch: [-128,127]
      | Yaw: [-128,127]
      | While these are controlled by sliders currently they
      | could be controlled by a user using twin analog joysticks
      | or by another intelligent system directing flight.
      | To make a system that balances itself we could use
      | readings off the 9-axis gyro to inform the system to
      | lean in the opposite direction.
  x_state : Inport
  Attitude Controller : Subsystem
  Bus Creator : BusCreator  Inputs=3
  Bus Selector1 : BusSelector  OutputSignals=phi,phi_dot,theta,theta_dot,psi,psi_dot,x,x_dot,y,y_dot,z,z_dot
  Heading Controller : Subsystem
  Motorspeeds : fuzblock/Fuzzy Logic  Controller  FIS=FuzzyMotorspeed  OutputSampleNumber=101  DataType=double  FuzzifiedInputs=off  RuleFiringStrengths=off  RuleOutputs=off  AggregatedOutputs=off  SimulateUsing=Interpreted execution  OutOfRangeInputValueMessage=warning  NoRuleFiredMessage=warning  EmptyOutputFuzzySetMessage=warning
  Saturation1 : Saturate  UpperLimit=255  LowerLimit=0  OutMin=[0]  OutMax=[255]
  Scope4 : Scope  NumInputPorts=4
  Subsystem : Subsystem
  Thrust Controller : Subsystem
  motorspeeds : Outport
  wires:
  Bus Selector1/9 -> ?  "<y>"
  Bus Creator/1 -> Motorspeeds/1
  Bus Selector1/8 -> ?  "<x_dot>"
  x_state/1 -> Bus Selector1/1
  Bus Selector1/7 -> ?  "<x>"
  Bus Selector1/10 -> ?  "<y_dot>"
  Bus Selector1/11 -> ?  "<z>"
  Attitude Controller/1(Desired Roll1) -> Bus Creator/1, Scope4/2  "Desired Roll"
  Attitude Controller/2(Desired Pitch1) -> Bus Creator/2, Scope4/3  "Desired Pitch"
  Bus Selector1/1 -> Attitude Controller/1(<phi>)  "<phi>"
  Bus Selector1/2 -> Attitude Controller/2(<phi_dot>)  "<phi_dot>"
  Bus Selector1/3 -> Attitude Controller/3(<theta>)  "<theta>"
  Bus Selector1/4 -> Attitude Controller/4(<theta_dot>)  "<theta_dot>"
  Heading Controller/1(Desired Yaw1) -> Scope4/4, Bus Creator/3
  Bus Selector1/5 -> Heading Controller/1(<psi>)  "<psi>"
  Bus Selector1/6 -> Heading Controller/2(<psi_dot>)  "<psi_dot>"
  Bus Selector1/12 -> Thrust Controller/1(<z_dot>)  "<z_dot>"
  Thrust Controller/1(Desired Thrust1) -> Subsystem/2(In2), Scope4/1
  Motorspeeds/1 -> Subsystem/1(In1)
  Subsystem/1(Out1) -> motorspeeds/1

== system Quadcopter_State_model_Arduino/Fuzzy Simulation/Quadcopter Dynamics1 ==
  U1 : Inport
  U2 : Inport  Port=2
  U3 : Inport  Port=3
  U4 : Inport  Port=4
  Omega_R : Inport  Port=5
  Bus Creator : BusCreator  Inputs=12
  Rotational Subsystem : Subsystem
  Translational Subsystem 2.0 : Subsystem
  Translational Wind Engine : Subsystem
  X_State : Outport
  wires:
  Rotational Subsystem/5(psi) -> Translational Subsystem 2.0/4(psi), Translational Wind Engine/3(psi), Bus Creator/5  "psi"
  Rotational Subsystem/2(phi_dot) -> Bus Creator/2  "phi_dot"
  Rotational Subsystem/3(theta) -> Translational Subsystem 2.0/3(theta), Translational Wind Engine/2(theta), Bus Creator/3  "theta"
  Rotational Subsystem/1(phi) -> Translational Subsystem 2.0/2(phi), Translational Wind Engine/1(phi), Bus Creator/1  "phi"
  Rotational Subsystem/4(theta_dot) -> Bus Creator/4  "theta_dot"
  Bus Creator/1 -> X_State/1  "X_State"
  Rotational Subsystem/6(psi_dot) -> Bus Creator/6  "psi_dot"
  U4/1 -> Rotational Subsystem/3(U4)
  U3/1 -> Rotational Subsystem/2(U3)
  U2/1 -> Rotational Subsystem/1(U2)
  Omega_R/1 -> Rotational Subsystem/4(Omega_R)
  Translational Wind Engine/1(FWx) -> Translational Subsystem 2.0/5(FWx)
  Translational Wind Engine/2(FWy) -> Translational Subsystem 2.0/6(FWy)
  Translational Wind Engine/3(FWz) -> Translational Subsystem 2.0/7(FWz)
  U1/1 -> Translational Subsystem 2.0/1(U1)
  Translational Subsystem 2.0/1(x) -> Bus Creator/7  "x"
  Translational Subsystem 2.0/2(x_dot) -> Bus Creator/8  "x_dot"
  Translational Subsystem 2.0/3(y) -> Bus Creator/9  "y"
  Translational Subsystem 2.0/4(y_dot) -> Bus Creator/10  "y_dot"
  Translational Subsystem 2.0/5(z) -> Bus Creator/11  "z"
  Translational Subsystem 2.0/6(z_dot) -> Bus Creator/12  "z_dot"

== system Quadcopter_State_model_Arduino/Fuzzy Simulation/Relative Speed ==
  Omega_1 : Inport
  Omega_2 : Inport  Port=2
  Omega_3 : Inport  Port=3
  Omega_4 : Inport  Port=4
  Add4 : Sum  Inputs=-+-+
  Omega_R : Outport
  wires:
  Omega_1/1 -> Add4/1
  Add4/1 -> Omega_R/1  "Omega_R"
  Omega_2/1 -> Add4/2
  Omega_3/1 -> Add4/3
  Omega_4/1 -> Add4/4

== system Quadcopter_State_model_Arduino/Fuzzy Simulation/Sensors ==
  X_State : Inport
  Sampling : Subsystem
  X_State Sensor : Outport
  wires:
  X_State/1 -> Sampling/1(X_State)
  Sampling/1(X_State Sensor) -> X_State Sensor/1

== system Quadcopter_State_model_Arduino/PID Simulation/Control Panel ==
  note: Control Panel
  note: Enabling Results in
      | Simulation Lag
  Rocker Switch{,1..4} (5 alike) : RockerSwitchBlock
      settings: Values={{'Off', 'On'}, [0 1]}
  Slider : SliderBlock  ScaleMin=-50  ScaleMax=50
  Slider1 : SliderBlock  ScaleMin=-50  ScaleMax=50
  Slider2 : SliderBlock  ScaleMin=-50  ScaleMax=0
  Slider3 : SliderBlock  ScaleMin=-3.14  ScaleMax=3.14

== system Quadcopter_State_model_Arduino/PID Simulation/Controller_Subsystem ==
  note: Position
  note: Controller
  X_State : Inport
  " " : Subsystem
  Altitude Controller : Subsystem
  Bus Selector : BusSelector  OutputSignals=phi,phi_dot,theta,theta_dot,psi,psi_dot,x,x_dot,y,y_dot,z,z_dot
  Desired X Position : Constant  Value=13.9952
  Desired Y Position : Constant  Value=0
  Desired Yaw : Constant  Value=0
  Desired Z Position : Constant  Value=-9.913277511961724
  Heading Controller : Subsystem
  Sum : Sum  Inputs=|+-
  Sum3 : Sum  Inputs=|-+
  Sum4 : Sum  Inputs=|+-
  Sum5 : Sum  Inputs=|-+
  U1 : Outport
  U2 : Outport  Port=2
  U3 : Outport  Port=3
  U4 : Outport  Port=4
  wires:
  Heading Controller/1(U4) -> U4/1  "U4 (psi)"
  Sum4/1 -> " "/4(e_x)  "e_x"
  Sum5/1 -> " "/5(e_y)  "e_y"
  Altitude Controller/1(U1) -> U1/1  "U1 (Z)"
  X_State/1 -> Bus Selector/1
  Bus Selector/1 -> " "/1(phi)  "<phi>"
  Bus Selector/2 -> ?  "<phi_dot>"
  Bus Selector/3 -> " "/2(theta)  "<theta>"
  Bus Selector/4 -> ?  "<theta_dot>"
  Bus Selector/5 -> " "/3(psi), Sum3/1  "<psi>"
  Bus Selector/6 -> ?  "<psi_dot>"
  Bus Selector/7 -> Sum4/1  "<x>"
  Bus Selector/8 -> ?  "<x_dot>"
  Bus Selector/9 -> Sum5/1  "<y>"
  Bus Selector/10 -> ?  "<y_dot>"
  Bus Selector/11 -> Sum/1  "<z>"
  Bus Selector/12 -> ?  "<z_dot>"
  Desired Z Position/1 -> Sum/2  "z_d"
  Desired Y Position/1 -> Sum5/2
  Desired Yaw/1 -> Sum3/2
  Sum/1 -> Altitude Controller/1(e_z)
  Sum3/1 -> Heading Controller/1(e_psi)
  Desired X Position/1 -> Sum4/2
  " "/1(U3) -> U3/1
  " "/2(U2) -> U2/1

== system Quadcopter_State_model_Arduino/PID Simulation/Motor_speed ==
  U1 : Inport
  U2 : Inport  Port=2
  U3 : Inport  Port=3
  U4 : Inport  Port=4
  1/2kf : Gain  Gain=1/(2*kf)
  1/2kf_ : Gain  Gain=1/(2*kf)
  1/4kf : Gain  Gain=1/(4*kf)
  1/4km : Gain  Gain=1/(4*km)
  Add : Sum  Inputs=+++
  Add1 : Sum  Inputs=+--
  Add2 : Sum  Inputs=+-+
  Add3 : Sum  Inputs=++-
  Saturation{,1..3} (4 alike) : Saturate  UpperLimit=inf  LowerLimit=0  ZeroCross=off
  Sqrt{,1..3} (4 alike) : Sqrt
  Omega_1 : Outport
  Omega_2 : Outport  Port=2
  Omega_3 : Outport  Port=3
  Omega_4 : Outport  Port=4
  wires:
  Sqrt/1 -> Omega_1/1  "Omega_1"
  Sqrt2/1 -> Omega_3/1  "Omega_3"
  1/4km/1 -> Add3/3, Add1/3, Add/3, Add2/3
  1/2kf_/1 -> Add/2, Add2/2
  Sqrt3/1 -> Omega_4/1  "Omega_4"
  1/4kf/1 -> Add/1, Add3/1, Add2/1, Add1/1
  1/2kf/1 -> Add3/2, Add1/2
  Sqrt1/1 -> Omega_2/1  "Omega_2"
  U3/1 -> 1/2kf_/1
  U4/1 -> 1/4km/1
  U2/1 -> 1/2kf/1
  U1/1 -> 1/4kf/1
  Add/1 -> Saturation/1  "Omega_1_sq"
  Saturation/1 -> Sqrt/1
  Saturation1/1 -> Sqrt1/1
  Add1/1 -> Saturation1/1  "Omega_2_sq"
  Saturation2/1 -> Sqrt2/1
  Add2/1 -> Saturation2/1  "Omega_3_sq"
  Saturation3/1 -> Sqrt3/1
  Add3/1 -> Saturation3/1  "Omega_4_sq"

== system Quadcopter_State_model_Arduino/PID Simulation/Quadcopter Dynamics ==
  U1 : Inport
  U2 : Inport  Port=2
  U3 : Inport  Port=3
  U4 : Inport  Port=4
  Omega_R : Inport  Port=5
  Bus Creator : BusCreator  Inputs=12
  Rotational Subsystem : Subsystem
  Translational Subsystem 2.0 : Subsystem
  Translational Wind Engine : Subsystem
  X_State : Outport
  wires:
  Rotational Subsystem/5(psi) -> Translational Subsystem 2.0/4(psi), Translational Wind Engine/3(psi), Bus Creator/5  "psi"
  Rotational Subsystem/2(phi_dot) -> Bus Creator/2  "phi_dot"
  Rotational Subsystem/3(theta) -> Translational Subsystem 2.0/3(theta), Translational Wind Engine/2(theta), Bus Creator/3  "theta"
  Rotational Subsystem/1(phi) -> Translational Subsystem 2.0/2(phi), Translational Wind Engine/1(phi), Bus Creator/1  "phi"
  Rotational Subsystem/4(theta_dot) -> Bus Creator/4  "theta_dot"
  Bus Creator/1 -> X_State/1  "X_State"
  Rotational Subsystem/6(psi_dot) -> Bus Creator/6  "psi_dot"
  U4/1 -> Rotational Subsystem/3(U4)
  U3/1 -> Rotational Subsystem/2(U3)
  U2/1 -> Rotational Subsystem/1(U2)
  Omega_R/1 -> Rotational Subsystem/4(Omega_R)
  Translational Wind Engine/1(FWx) -> Translational Subsystem 2.0/5(FWx)
  Translational Wind Engine/2(FWy) -> Translational Subsystem 2.0/6(FWy)
  Translational Wind Engine/3(FWz) -> Translational Subsystem 2.0/7(FWz)
  U1/1 -> Translational Subsystem 2.0/1(U1)
  Translational Subsystem 2.0/1(x) -> Bus Creator/7  "x"
  Translational Subsystem 2.0/2(x_dot) -> Bus Creator/8  "x_dot"
  Translational Subsystem 2.0/3(y) -> Bus Creator/9  "y"
  Translational Subsystem 2.0/4(y_dot) -> Bus Creator/10  "y_dot"
  Translational Subsystem 2.0/5(z) -> Bus Creator/11  "z"
  Translational Subsystem 2.0/6(z_dot) -> Bus Creator/12  "z_dot"

== system Quadcopter_State_model_Arduino/PID Simulation/Relative Speed ==
  Omega_1 : Inport
  Omega_2 : Inport  Port=2
  Omega_3 : Inport  Port=3
  Omega_4 : Inport  Port=4
  Add4 : Sum  Inputs=-+-+
  Omega_R : Outport
  wires:
  Omega_1/1 -> Add4/1
  Add4/1 -> Omega_R/1  "Omega_R"
  Omega_2/1 -> Add4/2
  Omega_3/1 -> Add4/3
  Omega_4/1 -> Add4/4

== system Quadcopter_State_model_Arduino/PID Simulation/Sensors ==
  X_State : Inport
  Enable Sensor Delay : Constant  Value=0
  Enable Sensor Noise : Constant  Value=0
  Noise Generator : Subsystem
  Sampling : Subsystem
  Switch : Switch  Criteria=u2 > Threshold  SaturateOnIntegerOverflow=off  InputSameDT=off
  Switch1 : Switch  Criteria=u2 > Threshold  SaturateOnIntegerOverflow=off  InputSameDT=off
  X_State Sensor : Outport
  wires:
  X_State/1 -> Sampling/1(X_State), Switch/3
  Switch/1 -> Noise Generator/1(X_State), Switch1/3
  Switch1/1 -> X_State Sensor/1
  Noise Generator/1(X_State_Noisy) -> Switch1/1
  Sampling/1(X_State Sensor) -> Switch/1
  Enable Sensor Delay/1 -> Switch/2
  Enable Sensor Noise/1 -> Switch1/2

== system Quadcopter_State_model_Arduino/PID Simulation/Visualization ==
  X_State : Inport
  Bus Creator1 : BusCreator  Inputs=3
  Bus Selector1 : BusSelector  OutputSignals=phi,phi_dot,theta,theta_dot,psi,psi_dot,x,x_dot,y,y_dot,z,z_dot
  Gain : Gain
  Gain1 : Gain  Gain=-1
  Gain2 : Gain
  Gain3 : Gain  Gain=-1
  Gain4 : Gain  Gain=-1
  Inertal to body frame : MATLAB Function  TreatAsAtomicUnit=on
  Rotation Matrix to VRML Rotation1 : vrlib/Utilities/Rotation Matrix to VR Rotation  maxzero=1e-12
  VR Sink : vrlib/VR Sink  InstantiateOnLoad=on  SampleTime=0.1  ViewEnable=on  RemoteChange=off  RemoteView=off  FieldsWritten=Wall_Mat.diffuseColor.3.1.1.double#Window_Mat.transparency.1.1.1.double#Landing_Mat.diffuseColor.3.1.1.double#Pole_1.Color.3.1.1.double#UAV.rotation.4.1.1.double#UAV.translation.3.1.1.double#HUDText1.string.1.-1.1.char  WorldFileName=uav_scene_drone_example.wrl  WorldDescription=UAV Competition Scene  AutoView=off  VideoDimensions=[]  AllowVariableSize=off  FigureProperties=[]
  wires:
  Bus Selector1/4 -> ?  "<theta_dot>"
  Bus Selector1/10 -> ?  "<y_dot>"
  X_State/1 -> Bus Selector1/1
  Bus Creator1/1 -> VR Sink/6  "X_State"
  Bus Selector1/2 -> ?  "<phi_dot>"
  Inertal to body frame/1(R) -> Rotation Matrix to VRML Rotation1/1
  ? -> VR Sink/7
  Rotation Matrix to VRML Rotation1/1 -> VR Sink/5
  ? -> VR Sink/4
  Bus Selector1/6 -> ?  "<psi_dot>"
  Bus Selector1/8 -> ?  "<x_dot>"
  Bus Selector1/12 -> ?  "<z_dot>"
  ? -> VR Sink/1
  ? -> VR Sink/2
  ? -> VR Sink/3
  Bus Selector1/11 -> Gain1/1  "<z>"
  Bus Selector1/9 -> Gain/1  "<y>"
  Bus Selector1/3 -> Gain3/1  "<theta>"
  Bus Selector1/5 -> Gain4/1  "<psi>"
  Bus Selector1/1 -> Inertal to body frame/3(psi)  "<phi>"
  Gain/1 -> Bus Creator1/1
  Gain1/1 -> Bus Creator1/2
  Bus Selector1/7 -> Gain2/1  "<x>"
  Gain2/1 -> Bus Creator1/3
  Gain3/1 -> Inertal to body frame/1(phi)
  Gain4/1 -> Inertal to body frame/2(theta)

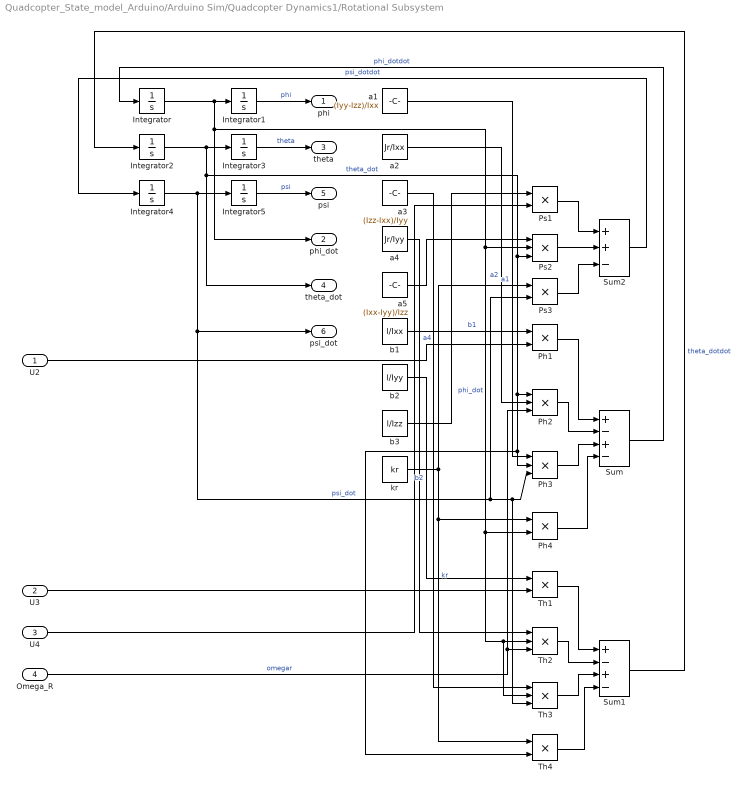
== system Quadcopter_State_model_Arduino/Arduino Sim/Quadcopter Dynamics1/Rotational Subsystem ==
  U2 : Inport
  U3 : Inport  Port=2
  U4 : Inport  Port=3
  Omega_R : Inport  Port=4
  Integrator{,1..5} (6 alike) : Integrator
  Ph1 : Product
  Ph2 : Product  Inputs=3
  Ph3 : Product  Inputs=3
  Ph4 : Product
  Ps1 : Product
  Ps2 : Product  Inputs=3
  Ps3 : Product
  Sum : Sum  Inputs=+-+-
  Sum1 : Sum  Inputs=+-+-
  Sum2 : Sum  Inputs=++-
  Th1 : Product
  Th2 : Product  Inputs=3
  Th3 : Product  Inputs=3
  Th4 : Product
  a1 : Constant  Value=(Iyy-Izz)/Ixx
  a2 : Constant  Value=Jr/Ixx
  a3 : Constant  Value=(Izz-Ixx)/Iyy
  a4 : Constant  Value=Jr/Iyy
  a5 : Constant  Value=(Ixx-Iyy)/Izz
  b1 : Constant  Value=l/Ixx
  b2 : Constant  Value=l/Iyy
  b3 : Constant  Value=l/Izz
  kr : Constant  Value=kr
  phi : Outport
  phi_dot : Outport  Port=2
  theta : Outport  Port=3
  theta_dot : Outport  Port=4
  psi : Outport  Port=5
  psi_dot : Outport  Port=6
  wires:
  U4/1 -> Ps1/2
  Ph3/1 -> Sum/3
  kr/1 -> Ps3/1, Ph4/1, Th4/1  "kr"
  Th1/1 -> Sum1/1
  Sum/1 -> Integrator/1  "phi_dotdot"
  Omega_R/1 -> Ph2/3, Th2/3  "omegar"
  Th2/1 -> Sum1/2
  Integrator4/1 -> Integrator5/1, psi_dot/1, Ps3/2, Th3/3, Ph3/3  "psi_dot"
  Integrator2/1 -> Integrator3/1, theta_dot/1, Ps2/3, Ph3/2, Th4/2, Ph2/1  "theta_dot"
  Th3/1 -> Sum1/3
  a4/1 -> Th2/1  "a4"
  Sum2/1 -> Integrator4/1  "psi_dotdot"
  Integrator1/1 -> phi/1  "phi"
  U2/1 -> Ph1/2
  Sum1/1 -> Integrator2/1  "theta_dotdot"
  Integrator/1 -> phi_dot/1, Ps2/2, Ph4/2, Th3/2, Th2/2, Integrator1/1  "phi_dot"
  Th4/1 -> Sum1/4
  Integrator3/1 -> theta/1  "theta"
  b1/1 -> Ph1/1  "b1"
  a3/1 -> Th3/1
  b3/1 -> Ps1/1
  a2/1 -> Ph2/2  "a2"
  a1/1 -> Ph3/1  "a1"
  a5/1 -> Ps2/1
  U3/1 -> Th1/2
  Ps3/1 -> Sum2/3
  Ps1/1 -> Sum2/1
  Ps2/1 -> Sum2/2
  Ph4/1 -> Sum/4
  b2/1 -> Th1/1  "b2"
  Ph1/1 -> Sum/1
  Ph2/1 -> Sum/2
  Integrator5/1 -> psi/1  "psi"

== system Quadcopter_State_model_Arduino/Arduino Sim/Quadcopter Dynamics1/Translational Subsystem 2.0 ==
  U1 : Inport
  phi : Inport  Port=2
  theta : Inport  Port=3
  psi : Inport  Port=4
  FWx : Inport  Port=5
  FWy : Inport  Port=6
  FWz : Inport  Port=7
  Integrator{6..11} (6 alike) : Integrator
  x_dotdot : Subsystem
      settings: PortSchema="{\"entries\":[{\"content\":{\"sides\":[{\"content\":{\"connectorIds\":[\"In1\",\"In2\",\"In3\",\"In4\",\"In5\",\"In6\",\"In7\"]},\"type\":\"ConnectorPlacement.EquallySpacedRectSide\",\"uuid\":\"e18be740-6f58-4938-bfd9-cb9ac7dcd4da\"},{\"content\":{\"connectorIds\":[\"In8\",\"Out1\"],\"side\":\"RIGHT\"},\"type\":\"ConnectorPlacement.EquallySpacedRectSide\",\"uuid\":\"68bb1cbd-6e96-465a-bd08-5b84ec49c8af\"},{\"content\":{\"connectorIds\":[],\"side\":\"TOP\"},\"type\":\"ConnectorPlacement.EquallySpacedRectSide\",\"uuid\":\"38ea75c0-d618-4b9d-8119-0da292fc369a\"}]},\"type\":\"ConnectorPlacement.EquallySpacedConnector\",\"uuid\":\"3f5248e6-8959-4c7a-b37c-028caf22ec16\"}],\"packageUris\":[\"http://schema.mathworks.com/mf0/Connector/R2020b\"],\"version\":\"1.0\"}"
  y_dotdot : Subsystem
      settings: PortSchema="{\"entries\":[{\"content\":{\"sides\":[{\"content\":{\"connectorIds\":[\"In1\",\"In2\",\"In3\",\"In4\",\"In5\",\"In6\",\"In7\"]},\"type\":\"ConnectorPlacement.EquallySpacedRectSide\",\"uuid\":\"e18be740-6f58-4938-bfd9-cb9ac7dcd4da\"},{\"content\":{\"connectorIds\":[\"In8\",\"Out1\"],\"side\":\"RIGHT\"},\"type\":\"ConnectorPlacement.EquallySpacedRectSide\",\"uuid\":\"68bb1cbd-6e96-465a-bd08-5b84ec49c8af\"},{\"content\":{\"connectorIds\":[],\"side\":\"TOP\"},\"type\":\"ConnectorPlacement.EquallySpacedRectSide\",\"uuid\":\"38ea75c0-d618-4b9d-8119-0da292fc369a\"}]},\"type\":\"ConnectorPlacement.EquallySpacedConnector\",\"uuid\":\"3f5248e6-8959-4c7a-b37c-028caf22ec16\"}],\"packageUris\":[\"http://schema.mathworks.com/mf0/Connector/R2020b\"],\"version\":\"1.0\"}"
  z_dodot : Subsystem
      settings: PortSchema="{\"entries\":[{\"content\":{\"sides\":[{\"content\":{\"connectorIds\":[\"In1\",\"In2\",\"In3\",\"In4\",\"In5\",\"In6\"]},\"type\":\"ConnectorPlacement.EquallySpacedRectSide\",\"uuid\":\"469c81c2-5293-4bed-8306-2e0ffdc3049a\"},{\"content\":{\"connectorIds\":[\"In7\",\"Out1\"],\"side\":\"RIGHT\"},\"type\":\"ConnectorPlacement.EquallySpacedRectSide\",\"uuid\":\"eb4ccd77-d780-4218-b458-09af15aced4a\"},{\"content\":{\"connectorIds\":[],\"side\":\"TOP\"},\"type\":\"ConnectorPlacement.EquallySpacedRectSide\",\"uuid\":\"6490e6c2-4333-4700-a2fe-e5c918a55a4d\"}]},\"type\":\"ConnectorPlacement.EquallySpacedConnector\",\"uuid\":\"88d53b3a-6da6-4ffe-908b-5dd465569eed\"}],\"packageUris\":[\"http://schema.mathworks.com/mf0/Connector/R2020b\"],\"version\":\"1.0\"}"
  x : Outport
  x_dot : Outport  Port=2
  y : Outport  Port=3
  y_dot : Outport  Port=4
  z : Outport  Port=5
  z_dot : Outport  Port=6
  wires:
  Integrator10/1 -> z_dot/1, z_dodot/7(z_dot), Integrator11/1  "z_dot"
  Integrator8/1 -> Integrator9/1, y_dotdot/8(y_dot), y_dot/1  "y_dot"
  Integrator9/1 -> y/1  "y"
  Integrator7/1 -> x/1  "x"
  Integrator6/1 -> x_dotdot/8(x_dot), x_dot/1, Integrator7/1  "x_dot"
  Integrator11/1 -> z/1  "z"
  U1/1 -> z_dodot/1(U1), y_dotdot/1(U1), x_dotdot/1(U1)  "U1"
  phi/1 -> y_dotdot/2(phi), x_dotdot/2(phi), z_dodot/2(phi)  "Phi"
  theta/1 -> z_dodot/3(theta), y_dotdot/3(theta), x_dotdot/3(theta)  "Theta"
  psi/1 -> y_dotdot/4(psi), x_dotdot/4(psi)  "Psi"
  FWx/1 -> z_dodot/4(FWx), y_dotdot/5(FWx), x_dotdot/5(FWx)  "FWx"
  FWy/1 -> z_dodot/5(FWy), y_dotdot/6(FWy), x_dotdot/6(FWy)  "FWy"
  FWz/1 -> z_dodot/6(FWz), y_dotdot/7(FWz), x_dotdot/7(FWz)  "FWz"
  z_dodot/1(z_dotdot) -> Integrator10/1
  y_dotdot/1(y_dotdot) -> Integrator8/1
  x_dotdot/1(x_dotdot) -> Integrator6/1

== system Quadcopter_State_model_Arduino/Arduino Sim/Quadcopter Dynamics1/Translational Wind Engine ==
  phi : Inport
  theta : Inport  Port=2
  psi : Inport  Port=3
  Projected Areas : Subsystem
  Wind Forces : Subsystem
  Wind Generation : Subsystem
  FWx : Outport
  FWy : Outport  Port=2
  FWz : Outport  Port=3
  wires:
  theta/1 -> Projected Areas/1(theta)
  Wind Generation/3(VWz) -> Wind Forces/6(VWz)
  Projected Areas/3(Az) -> Wind Forces/3(Az)
  Wind Forces/3(FWz) -> FWz/1
  Wind Generation/2(VWy) -> Wind Forces/5(VWy)
  Projected Areas/1(Ax) -> Wind Forces/1(Ax)
  Projected Areas/2(Ay) -> Wind Forces/2(Ay)
  Wind Generation/1(VWx) -> Wind Forces/4(VWx)
  phi/1 -> Projected Areas/3(phi)
  psi/1 -> Projected Areas/2(psi)
  Wind Forces/2(FWy) -> FWy/1
  Wind Forces/1(FWx) -> FWx/1

== system Quadcopter_State_model_Arduino/Board Fuzzy Only/Fuzzy Control System/Attitude Controller ==
  <phi> : Inport
  <phi_dot> : Inport  Port=2
  <theta> : Inport  Port=3
  <theta_dot> : Inport  Port=4
  Bus Creator1 : BusCreator  Inputs=4
  Demux1 : Demux  Outputs=2
  Desired Pitch2 : Constant  Value=Desired_Pitch
  Desired Roll2 : Constant  Value=Desired_Roll
  DesiredPitchRoll : fuzblock/Fuzzy Logic  Controller  FIS=DesiredPitchRoll  OutputSampleNumber=101  DataType=double  FuzzifiedInputs=off  RuleFiringStrengths=off  RuleOutputs=off  AggregatedOutputs=off  SimulateUsing=Interpreted execution  OutOfRangeInputValueMessage=warning  NoRuleFiredMessage=warning  EmptyOutputFuzzySetMessage=warning
  Sum1 : Sum  Inputs=|-+
  Sum2 : Sum  Inputs=|-+
  e_pitch_sat : Saturate  UpperLimit=0.3  LowerLimit=-0.3  OutMin=[-0.3]  OutMax=[0.3]
  e_roll_sat : Saturate  UpperLimit=0.3  LowerLimit=-0.3  OutMin=[-0.3]  OutMax=[0.3]
  phidot_sat1 : Saturate  UpperLimit=0.3  LowerLimit=-0.3  OutMin=[-0.3]  OutMax=[0.3]
  thetadot_sat : Saturate  UpperLimit=0.3  LowerLimit=-0.3  OutMin=[-0.3]  OutMax=[0.3]
  Desired Roll1 : Outport
  Desired Pitch1 : Outport  Port=2
  wires:
  e_roll_sat/1 -> Bus Creator1/1
  phidot_sat1/1 -> Bus Creator1/4
  Sum2/1 -> e_pitch_sat/1  "e_pitch"
  Desired Roll2/1 -> Sum1/2
  e_pitch_sat/1 -> Bus Creator1/2
  DesiredPitchRoll/1 -> Demux1/1
  Bus Creator1/1 -> DesiredPitchRoll/1
  Demux1/2 -> Desired Pitch1/1  "Desired Pitch"
  Desired Pitch2/1 -> Sum2/2
  Sum1/1 -> e_roll_sat/1  "e_roll"
  thetadot_sat/1 -> Bus Creator1/3
  <phi>/1 -> Sum2/1
  <theta>/1 -> Sum1/1
  Demux1/1 -> Desired Roll1/1  "Desired Roll"
  <phi_dot>/1 -> phidot_sat1/1
  <theta_dot>/1 -> thetadot_sat/1
